simulink model "bumplessTransfer2"  (R2019a)
settings: Solver=VariableStepAuto  StartTime=0.0  StopTime=30  RelTol=1e-3
values from neighbouring files (symbols this model uses):
  Ki = 2    [mainAntiWindup1.m]    (also in mainAntiWindup2.m; mainBumpless.m; mainLimAzioneDerivativa.m = 1; mainWindupIntegrale.m)
  Kp = 2    [mainAntiWindup1.m]    (also in mainAntiWindup2.m; mainBumpless.m; mainLimAzioneDerivativa.m; mainWindupIntegrale.m = 0)
  tswitch = 10    [mainBumpless.m]
  uman = 1    [mainBumpless.m]
settings Model: Creator=adria  LastModifiedBy=adria

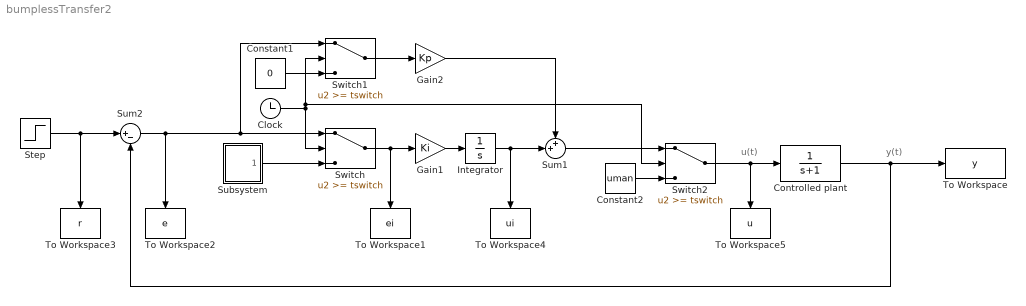
== system bumplessTransfer2 ==
  note: u(t)
  note: y(t)
  Clock : Clock
  Constant1 : Constant  Value=0
  Constant2 : Constant  Value=uman
  Controlled plant : TransferFcn  Denominator=[1 1]
  Gain1 : Gain  Gain=Ki
  Gain2 : Gain  Gain=Kp
  Integrator : Integrator
  Step : Step  SampleTime=0
  Subsystem : Subsystem
  Sum1 : Sum  Inputs=++|
  Sum2 : Sum  Inputs=|+-
  Switch : Switch  Threshold=tswitch
  Switch1 : Switch  Threshold=tswitch
  Switch2 : Switch  Threshold=tswitch
  To Workspace : ToWorkspace  VariableName=y  SaveFormat=Structure With Time  SampleTime=-1
  To Workspace1 : ToWorkspace  VariableName=ei  SaveFormat=Structure With Time  SampleTime=-1
  To Workspace2 : ToWorkspace  VariableName=e  SaveFormat=Structure With Time  SampleTime=-1
  To Workspace3 : ToWorkspace  VariableName=r  SaveFormat=Structure With Time  SampleTime=-1
  To Workspace4 : ToWorkspace  VariableName=ui  SaveFormat=Structure With Time  SampleTime=-1
  To Workspace5 : ToWorkspace  VariableName=u  SaveFormat=Structure With Time  SampleTime=-1
  wires:
  Step/1 -> To Workspace3/1, Sum2/1
  Integrator/1 -> Sum1/2, To Workspace4/1
  Gain1/1 -> Integrator/1
  Controlled plant/1 -> To Workspace/1, Sum2/2
  Sum2/1 -> To Workspace2/1, Switch1/1, Switch/1
  Gain2/1 -> Sum1/1
  Switch/1 -> To Workspace1/1, Gain1/1
  Subsystem/1("uman ") -> Switch/3
  Switch1/1 -> Gain2/1
  Constant1/1 -> Switch1/3
  Clock/1 -> Switch1/2, Switch2/2, Switch/2
  Constant2/1 -> Switch2/3
  Sum1/1 -> Switch2/1
  Switch2/1 -> Controlled plant/1, To Workspace5/1

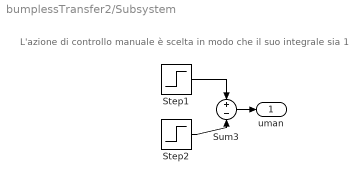
== system bumplessTransfer2/Subsystem ==
  note: L'azione di controllo manuale è scelta in modo che il suo integrale sia 1
  Step1 : Step  Time=0  After=1/Kp  SampleTime=0
  Step2 : Step  After=1/Kp  SampleTime=0
  Sum3 : Sum  Inputs=+-
  "uman " : Outport
  wires:
  Step1/1 -> Sum3/1
  Step2/1 -> Sum3/2
  Sum3/1 -> "uman "/1
